simulink model "StateflowBlock"  (R2024a)
settings: Solver=FixedStepDiscrete  StartTime=0.0  StopTime=Inf  FixedStep=0.1  RelTol=1e-3
settings Model: TunableVars=kp,PWMsl_l,PWMsl_r,PWMsr_l,PWMsr_r  TunableVarsStorageClass=Auto,Auto,Auto,Auto,Auto  TunableVarsTypeQualifier=,,,,  Creator=omars  LastModifiedBy=lukas
settings DataIOCC: ReturnWorkspaceOutputs=off
settings OptimizationCC: EnhancedBackFolding=on  PassReuseOutputArgsAs=Individual arguments  ZeroExternalMemoryAtStartup=off  ZeroInternalMemoryAtStartup=off  OptimizeBlockOrder=speed  DifferentSizesBufferReuse=on  OptimizationCustomize=off  EfficientTunableParamExpr=on
settings DebuggingCC: ParameterTunabilityLossMsg=error
settings SFSimCC: MATLABDynamicMemAlloc=off
settings RTWCC: Description=Embedded Coder  SystemTargetFile=ert.tlc  GenCodeOnly=on  TemplateMakefile=ert_default_tmf  GPUComputeCapability=3.5
settings CodeAppCC: ForceParamTrailComments=on  IgnoreCustomStorageClasses=off  OperatorAnnotations=on  SimulinkDataObjDesc=on  SFDataObjDesc=on  InsertBlockDesc=on
settings ERTTargetCC: TargetLangStandard=C99 (ISO)  ERTCustomFileTemplate=example_file_process.tlc

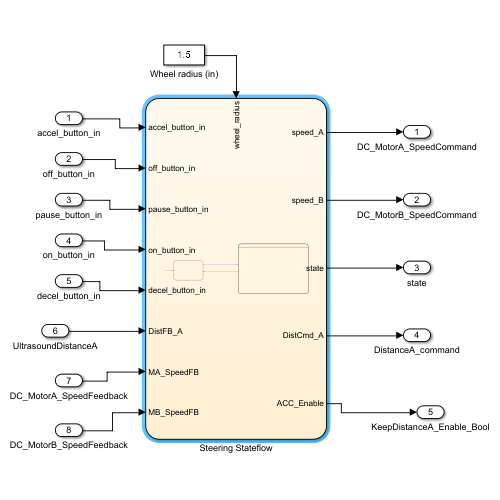
[thumbnail: Simulink's stored preview of the top-level diagram]
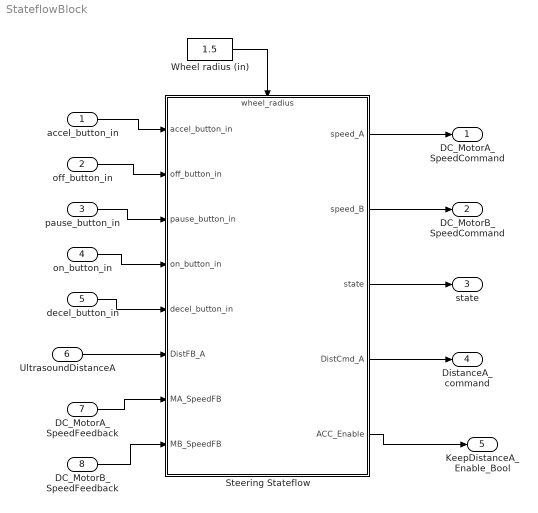
== system StateflowBlock ==
  accel_button_in : Inport
  off_button_in : Inport  Port=2
  pause_button_in : Inport  Port=3
  on_button_in : Inport  Port=4
  decel_button_in : Inport  Port=5
  UltrasoundDistanceA : Inport  Port=6
  DC_MotorA_SpeedFeedback : Inport  Port=7
  DC_MotorB_SpeedFeedback : Inport  Port=8
  Steering Stateflow : Stateflow chart  TreatAsAtomicUnit=on
      settings: PortSchema="{\"entries\":[{\"content\":{\"sides\":[{\"content\":{\"connectorIds\":[\"In3\",\"In4\",\"In5\",\"In6\",\"In9\",\"In1\",\"In7\",\"In8\"]},\"type\":\"ConnectorPlacement.EquallySpacedRectSide\",\"uuid\":\"80dcc8d6-aa19-4329-80f2-43be3f76ecea\"},{\"content\":{\"connectorIds\":[\"Out2\",\"Out3\",\"Out5\",\"Out4\",\"Out1\"],\"side\":\"RIGHT\"},\"type\":\"ConnectorPlacement.EquallySpacedRectSide\",\"uuid\":\"4e6e0fce-41ed-43d9-af05-514bba8f8dbd\"},{\"content\":{\"connectorIds\":[\"In2\"],\"side\":\"TOP\"},\"type\":\"ConnectorPlacement.EquallySpacedRectSide\",\"uuid\":\"7ace72f0-dafc-45ef-b347-5f7d59858afe\"},{\"content\":{\"side\":\"BOTTOM\"},\"type\":\"ConnectorPlacement.EquallySpacedRectSide\",\"uuid\":\"573fd0e0-7faf-456f-ae2d-765ad0ec4cd5\"}]},\"type\":\"ConnectorPlacement.EquallySpacedConnector\",\"uuid\":\"0e6ea89e-5511-46b0-968b-5e141f0ce0a1\"}],\"packageUris\":[\"http://schema.mathworks.com/mf0/Connector/R2020b\"],\"version\":\"1.0\"}"
  Wheel radius (in) : Constant  Value=1.5
  DC_MotorA_SpeedCommand : Outport
  DC_MotorB_SpeedCommand : Outport  Port=2
  state : Outport  Port=3
  DistanceA_command : Outport  Port=4
  KeepDistanceA_Enable_Bool : Outport  Port=5
  wires:
  pause_button_in/1 -> Steering Stateflow/5(pause_button_in)
  Steering Stateflow/3(speed_B) -> DC_MotorB_SpeedCommand/1
  Steering Stateflow/5(state) -> state/1
  Steering Stateflow/2(speed_A) -> DC_MotorA_SpeedCommand/1
  off_button_in/1 -> Steering Stateflow/4(off_button_in)
  accel_button_in/1 -> Steering Stateflow/3(accel_button_in)
  decel_button_in/1 -> Steering Stateflow/9(decel_button_in)
  on_button_in/1 -> Steering Stateflow/6(on_button_in)
  Wheel radius (in)/1 -> Steering Stateflow/2(wheel_radius)
  Steering Stateflow/4(DistCmd_A) -> DistanceA_command/1
  Steering Stateflow/1(ACC_Enable) -> KeepDistanceA_Enable_Bool/1
  UltrasoundDistanceA/1 -> Steering Stateflow/1(DistFB_A)
  DC_MotorB_SpeedFeedback/1 -> Steering Stateflow/8(MB_SpeedFB)
  DC_MotorA_SpeedFeedback/1 -> Steering Stateflow/7(MA_SpeedFB)

== stateflow chart StateflowBlock/Steering Stateflow ==
  settings: updateMethod=DISCRETE  sampleTime=0.1
  state ON
    state Acceleration
      speed = speed + 3/wheel_radius;
      speed_A = speed;
      speed_B = -1*speed;
      state = 2;
    state Ada
      DistCmd_A = 100;
      state = 5;
      ACC_Enable = 1;
    state Running
      speed_A = speed;
      speed_B = -1*speed;
      state = 1;
      ACC_Enable = 0;
    state Pause
      speed_A = 0;
      speed_B = 0;
      state = 4;
      ACC_Enable = 0;
    state Deceleration
      speed = speed - 3/wheel_radius;
      speed_A = speed;
      speed_B = -1*speed;
      state = 3;
    note: Speed example : if you want the rover to move 6(in/sec)
        | You should put 6(in/sec) / 1.5(wheel radius) = 2 rad/sec
    Running -> Acceleration [order 2] : [accel_button_in > 0]
    Running -> Ada [order 4] : [DistFB_A < 200]
    Pause -> Acceleration [order 1] : [on_button_in > 0]
    Acceleration -> Running [order 2] : [accel_button_in == 0]
    Acceleration -> Pause [order 1] : [pause_button_in > 0]
    Ada -> Pause [order 2] : [DistFB_A > 250]
    Ada -> Pause [order 1] : [pause_button_in > 0]
    (default) -> Running
    Deceleration -> Running [order 1] : [decel_button_in == 0]
    Running -> Deceleration [order 1] : [decel_button_in > 0]
    Running -> Pause [order 3] : [pause_button_in > 0]
    Pause -> Running [order 2] : [on_button_in > 0]
    Pause -> Deceleration [order 3] : [on_button_in > 0]
    Deceleration -> Pause [order 2] : [pause_button_in > 0]
  state OFF
    speed = 0
    speed_A = -speed;
    speed_B = speed;
    state = 0;
    ACC_Enable = 0;
  OFF -> ON : [on_button_in > 0]
  (default) -> OFF
  ON -> OFF : [off_button_in > 0]
  data: DistFB_A input; ACC_Enable output; wheel_radius input; accel_button_in input boolean; off_button_in input boolean; speed_A output double; speed_B output double; DistCmd_A output; pause_button_in input boolean =500; state output; on_button_in input; MA_SpeedFB input; MB_SpeedFB input; decel_button_in input; speed local
